simulink library "lib6DOFDerivativeOfEquations"  (R2020b)
settings: Solver=VariableStepAuto  StartTime=0.0  StopTime=10.0  RelTol=1e-3
undefined symbols (not defined in the file): data
settings Model: Creator=caatay  LastModifiedBy=caatay

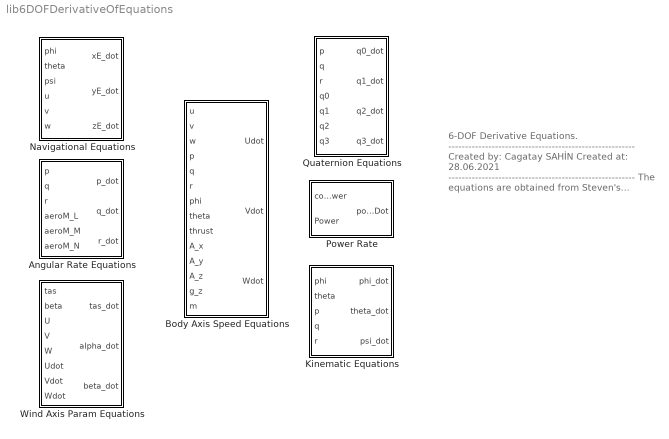
== system lib6DOFDerivativeOfEquations ==
  note: 6-DOF Derivative Equations.
      | --------------------------------------------------------
      | Created by: Cagatay SAHİN
      | Created at: 28.06.2021
      | --------------------------------------------------------
      | The equations are obtained from
      | Steven's textbook.
      | The reference book can be found in
      | "references folder".
      | --------------------------------------------------------
      | for question:
      | cagataysahin44@gmail.com
  Angular Rate Equations : Subsystem  mask(Equation of Motion - Derivative Equations of Motion - CAME (Angular Rate) Equations.){I_xx=data.acSpec.inertia.I_xx, I_yy=data.acSpec.inertia.I_yy, I_zz=data.acSpec.inertia.I_zz, I_xz=data.acSpec.inertia.I_xz, h_x=data.engine.specs.angMom.h_x}
      mask prompts: I_xx "Inertia on X-axis"; I_yy "Inertia on Y-axis"; I_zz "Inertia on Z-axis"; I_xz "Inertia on XZ-axis"; h_x "Angular Momentum on X-axis"
      mask help: Aircraft Conversation of Angular Momentum Equation which calculates angular rates.
      mask Help:
      | Aircraft Conversation of Angular Momentum Equation which calculates angular rates which using moment and state information as an input.
      | -------------------------------------------------------------------------------------------------------------------------------------------------
      | Inputs of this block:
      | 	Body Axis Speed: U, V, W information [ft/s].
      | 	Body Axis Moments: M_l, M_M, M_N information
      | Outputs of this block:
      | 	Ang. Rates Der.: Derivative of Angular Rates [rad/sec^2].
      | -------------------------------------------------------------------------------------------------------------------------------------------------
      | Equations that in this block can be found in Steven's textbook. This textbook is in "literature" subfolder.
      | for question: "cagataysahin44@gmail.com".
      mask Display:
      | port_label('input',1,'p','texmode','on');
      | port_label('input',2,'q','texmode','on');
      | port_label('input',3,'r','texmode','on');
      | port_label('input',4,'M_{L}','texmode','on');
      | port_label('input',5,'M_{M}','texmode','on');
      | port_label('input',6,'M_{N}','texmode','on');
      | 
      | port_label('output',1,'p_{der}','texmode','on');
      | port_label('output',2,'q_{der}','texmode','on');
      | port_label('output',3,'r_{der}','texmode','on');
  Body Axis Speed Equations : Subsystem  mask(EOM Model - Derivative Equation of Motion - Body Axis Speed Equations){}
      mask help: Aircraft body axis speeds calculation equations.
      mask Help:
      | This block can calculate aircraft's body axis speeds with using state, thrust, force and gravity information.
      | -------------------------------------------------------------------------------------------------------------------------------------------------
      | Inputs of this block:
      | 	Euler Angles: Roll, Pitch information [rad].
      | 	Body Axis Speed: U, V, W information [ft/s].
      | 	T: Thrust information [lbf].
      | 	A_{i}: Aerodynamic force information [lbf].
      | 	g: gravity information [ft/sec^2].
      | 	m: Aircraft Mass [slug].
      | Outputs of this block:
      | 	Body Axis Speed Ders. Derivative of body axis speeds [ft/sec^2].
      | -------------------------------------------------------------------------------------------------------------------------------------------------
      | Equations that in this block can be found in Steven's textbook. This textbook is in "literature" subfolder.
      | for question: "cagataysahin44@gmail.com".
      mask Display:
      | port_label('input',1,'U','texmode','on');
      | port_label('input',2,'V','texmode','on');
      | port_label('input',3,'W','texmode','on');
      | port_label('input',4,'p','texmode','on');
      | port_label('input',5,'q','texmode','on');
      | port_label('input',6,'r','texmode','on');
      | port_label('input',7,'\phi','texmode','on');
      | port_label('input',8,'\theta','texmode','on');
      | port_label('input',9,'T','texmode','on');
      | port_label('input',10,'A_{x}','texmode','on');
      | port_label('input',11,'A_{y}','texmode','on');
      | port_label('input',12,'A_{z}','texmode','on');
      | port_label('input',13,'g_{z}','texmode','on');
      | port_label('input',14,'m','texmode','on');
      | 
      | port_label('output',1,'U_{der}','texmode','on');
      | port_label('output',2,'V_{der}','texmode','on');
      | port_label('output',3,'W_{der}','texmode','on');
  Kinematic Equations : Subsystem  mask(Equation of Motion - Derivative Equation of Motion - Kinematic Equation for Euler Angles.){}
      mask help: Aircraft kinematic equtions which is in Euler Angles form.
      mask Help:
      | This block can calculate aircaft's kinematic parameters in Euler Angles form.
      | -------------------------------------------------------------------------------------------------------------------------------------------------
      | Inputs of this block:
      | 	Euler Angles: Roll, Pitch, information [rad].
      | 	Body Axis Angular Rates: p, q, r information [rad/s].
      | Outputs of this block:
      | 	Euler Angles Ders: Derivative of Euler Angles.
      | -------------------------------------------------------------------------------------------------------------------------------------------------
      | Equations that in this block can be found in Steven's textbook. This textbook is in "literature" subfolder.
      | for question: "cagataysahin44@gmail.com".
      mask Display:
      | port_label('input',1,'\phi','texmode','on');
      | port_label('input',2,'\theta','texmode','on');
      | port_label('input',3,'p','texmode','on');
      | port_label('input',4,'q','texmode','on');
      | port_label('input',5,'r','texmode','on');
      | 
      | port_label('output',1,'\phi_{der}','texmode','on');
      | port_label('output',2,'\theta_{der}','texmode','on');
      | port_label('output',3,'\psi_{der}','texmode','on');
  Navigational Equations : Subsystem  mask(EOM Model - Derivative Equations - Navigational Equations){}
      mask help: Aircraft navigational equations which is known as flight path.
      mask Help:
      | This block can calculate aircaft's flight path information with using state inputs.
      | -------------------------------------------------------------------------------------------------------------------------------------------------
      | Inputs of this block:
      | 	Euler Angles: Roll, Pitch, Yaw information [rad].
      | 	Body Axis Speed: U, V, W information [ft/s].
      | Outputs of this block:
      | 	p_{e}: Derivative of position of aircraft in NED Coordinate System [ft].
      | -------------------------------------------------------------------------------------------------------------------------------------------------
      | Equations that in this block can be found in Steven's textbook. This textbook is in "literature" subfolder.
      | for question: "cagataysahin44@gmail.com".
      mask Display:
      | port_label('input',1,'\phi','texmode','on');
      | port_label('input',2,'\theta','texmode','on');
      | port_label('input',3,'\psi','texmode','on');
      | port_label('input',4,'u','texmode','on');
      | port_label('input',5,'v','texmode','on');
      | port_label('input',6,'w','texmode','on');
      | 
      | port_label('output',1,'x_{e_{der}}','texmode','on');
      | port_label('output',2,'y_{e_{der}}','texmode','on');
      | port_label('output',3,'z_{e_{der}}','texmode','on');
  Power Rate : Subsystem  mask(EOM Model - Derivative of Equation of Motion - Power Rate Calculation){}
      mask help: Derivative of power calculation with using actual power information as a state and commanded power information from throttle command.
      mask Help:
      | This block can calculate aircaft's power derivative equation.
      | -------------------------------------------------------------------------------------------------------------------------------------------------
      | Inputs of this block:
      | 	cmdPow: Commanded Power [hp].
      | 	actPow: Actual Power [hp].
      | Outputs of this block:
      | 	powDot: Derivative of Power [hp/s]
      | -------------------------------------------------------------------------------------------------------------------------------------------------
      | Equations that in this block can be found in Steven's textbook. This textbook is in "literature" subfolder.
      | for question: "cagataysahin44@gmail.com".
      mask Display:
      | port_label('input',1,'Pow_{cmd}','texmode','on');
      | port_label('input',2,'Pow_{act}','texmode','on');
      | 
      | port_label('output',1,'der_{Pow_{act}}','texmode','on');
  Quaternion Equations : Subsystem  mask(Equation of Motion - Derivative Equation of Motion - Kinematic Equation for Quaternion Angles.){}
      mask help: Aircraft kinematic equtions which is in quaternion angles form.
      mask Help:
      | This block can calculate aircaft's kinematic parameters in quaternion angles form.
      | -------------------------------------------------------------------------------------------------------------------------------------------------
      | Inputs of this block:
      | 	Quaternion Angles: q0, q1, q2, q3, information [rad].
      | 	Body Axis Angular Rates: p, q, r information [rad/s].
      | Outputs of this block:
      | 	Quaternion Angles Ders: Derivative of Quaternion Angles.
      | -------------------------------------------------------------------------------------------------------------------------------------------------
      | Equations that in this block can be found in Steven's textbook. This textbook is in "literature" subfolder.
      | for question: "cagataysahin44@gmail.com".
      mask Display:
      | port_label('input',1,'p','texmode','on');
      | port_label('input',2,'q','texmode','on');
      | port_label('input',3,'r','texmode','on');
      | port_label('input',4,'q_{0}','texmode','on');
      | port_label('input',5,'q_{1}','texmode','on');
      | port_label('input',6,'q_{2}','texmode','on');
      | port_label('input',7,'q_{3}','texmode','on');
      | 
      | port_label('output',1,'q_{1_{der}}','texmode','on');
      | port_label('output',2,'q_{2_{der}}','texmode','on');
      | port_label('output',3,'q_{3_{der}}','texmode','on');
      | port_label('output',4,'q_{4_{der}}','texmode','on');
  Wind Axis Param Equations : Subsystem  mask(EOM Model - Derivative of Equation of Motion - Wind Axis Paramater Equations.){}
      mask help: Aircraft wind parameter information calculation which is angle of attack, angle of sideslip and true airspeed.
      mask Help:
      | This block can calculate aircaft's wind parameters which using state inputs.
      | -------------------------------------------------------------------------------------------------------------------------------------------------
      | Inputs of this block:
      | 	Wind Params: True airspeed, AoA and AoS [ft/s, rad].
      | 	Body Speeds: U, V, W information [ft/s].
      | 	Body Speed Ders: U, V, W derivative information [ft/sec^2].
      | Outputs of this block:
      | 	Wind Param Ders: Derivative information of wind parameters. [ft/sec^2, rad/sec].
      | -------------------------------------------------------------------------------------------------------------------------------------------------
      | Equations that in this block can be found in Steven's textbook. This textbook is in "literature" subfolder.
      | for question: "cagataysahin44@gmail.com".
      mask Display:
      | port_label('input',1,'V_{tas}','texmode','on');
      | port_label('input',2,'\beta','texmode','on');
      | port_label('input',3,'U','texmode','on');
      | port_label('input',4,'V','texmode','on');
      | port_label('input',5,'W','texmode','on');
      | port_label('input',6,'U_{der}','texmode','on');
      | port_label('input',7,'V_{der}','texmode','on');
      | port_label('input',8,'W_{der}','texmode','on');
      | 
      | port_label('output',1,'V_{tas_{der}}','texmode','on');
      | port_label('output',2,'\alpha_{der}','texmode','on');
      | port_label('output',3,'\beta_{der}','texmode','on');

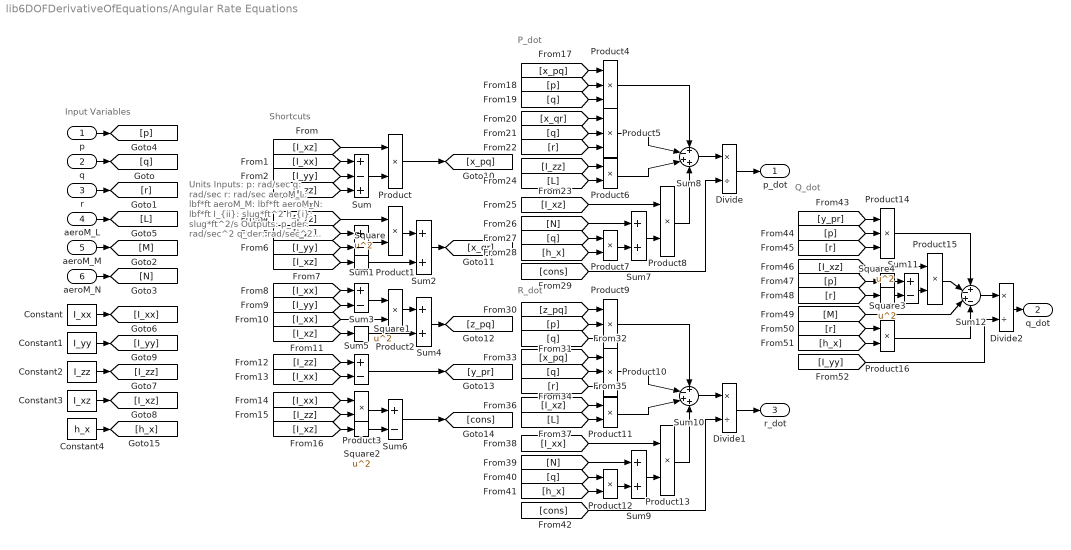
== system lib6DOFDerivativeOfEquations/Angular Rate Equations ==
  note: Q_dot
  note: P_dot
  note: Shortcuts
  note: Units
      | Inputs:
      | p: rad/sec
      | q: rad/sec
      | r: rad/sec
      | aeroM_L: lbf*ft
      | aeroM_M: lbf*ft
      | aeroM_N: lbf*ft
      | I_{ii}: slug*ft^2
      | h_{i}: slug*ft^2/s
      | Outputs:
      | p_der: rad/sec^2
      | q_der: rad/sec^2
      | r_der: rad/sec^2
  note: Input Variables
  note: R_dot
  p : Inport
  q : Inport  Port=2
  r : Inport  Port=3
  aeroM_L : Inport  Port=4
  aeroM_M : Inport  Port=5
  aeroM_N : Inport  Port=6
  Constant : Constant  Value=I_xx
  Constant1 : Constant  Value=I_yy
  Constant2 : Constant  Value=I_zz
  Constant3 : Constant  Value=I_xz
  Constant4 : Constant  Value=h_x
  Divide : Product  Inputs=*/
  Divide1 : Product  Inputs=*/
  Divide2 : Product  Inputs=*/
  Product{,1..3,6..8,11..13,15..16} (12 alike) : Product
  Product{4..5,9..10,14} (5 alike) : Product  Inputs=3
  Square{,1..4} (5 alike) : Math  Operator=square  SignedPower=on  SaturateOnIntegerOverflow=on
  Sum : Sum  Inputs=+-+
  Sum{1,3,5..6,11} (5 alike) : Sum  Inputs=+-
  Sum10 : Sum  Inputs=+-++
  Sum12 : Sum  Inputs=+-+-
  Sum{2,4,7,9} (4 alike) : Sum
  Sum8 : Sum  Inputs=+-++
  p_dot : Outport  VectorParamsAs1DForOutWhenUnconnected=off
  q_dot : Outport  Port=2  VectorParamsAs1DForOutWhenUnconnected=off
  r_dot : Outport  Port=3  VectorParamsAs1DForOutWhenUnconnected=off
  wires:
  p/1 -> [p]
  q/1 -> [q]
  r/1 -> [r]
  aeroM_L/1 -> [L]
  aeroM_M/1 -> [M]
  aeroM_N/1 -> [N]
  Constant/1 -> [I_xx]
  Constant3/1 -> [I_xz]
  Constant2/1 -> [I_zz]
  Constant1/1 -> [I_yy]
  [I_xx] -> Sum/1
  [I_zz] -> Sum/3
  [I_yy] -> Sum/2
  [I_xz] -> Product/1
  Sum/1 -> Product/2
  Product/1 -> [x_pq]
  [I_xz] -> Square/1
  [I_zz] -> Sum1/1
  [I_yy] -> Sum1/2
  Sum1/1 -> Product1/2
  [I_zz] -> Product1/1
  Product1/1 -> Sum2/1
  Square/1 -> Sum2/2
  Sum2/1 -> [x_qr]
  [I_xz] -> Square1/1
  [I_xx] -> Product2/2
  [I_yy] -> Sum3/2
  [I_xx] -> Sum3/1
  Sum3/1 -> Product2/1
  Product2/1 -> Sum4/1
  Square1/1 -> Sum4/2
  Sum4/1 -> [z_pq]
  [I_zz] -> Sum5/1
  [I_xx] -> Sum5/2
  Sum5/1 -> [y_pr]
  [I_zz] -> Product3/2
  [I_xx] -> Product3/1
  [I_xz] -> Square2/1
  Product3/1 -> Sum6/1
  Square2/1 -> Sum6/2
  Sum6/1 -> [cons]
  Constant4/1 -> [h_x]
  [x_pq] -> Product4/1
  [p] -> Product4/2
  [q] -> Product4/3
  [q] -> Product5/2
  [x_qr] -> Product5/1
  [r] -> Product5/3
  [I_zz] -> Product6/1
  [L] -> Product6/2
  [q] -> Product7/1
  [h_x] -> Product7/2
  [N] -> Sum7/1
  [I_xz] -> Product8/1
  Product7/1 -> Sum7/2
  Sum7/1 -> Product8/2
  Product6/1 -> Sum8/3
  Product5/1 -> Sum8/2
  Product4/1 -> Sum8/1
  Product8/1 -> Sum8/4
  Sum8/1 -> Divide/1
  Divide/1 -> p_dot/1
  [cons] -> Divide/2
  Product12/1 -> Sum9/2
  Sum9/1 -> Product13/2
  [N] -> Sum9/1
  Sum10/1 -> Divide1/1
  [q] -> Product12/1
  Product13/1 -> Sum10/4
  Product9/1 -> Sum10/1
  [I_xz] -> Product11/1
  [h_x] -> Product12/2
  Divide1/1 -> r_dot/1
  [x_pq] -> Product10/1
  [q] -> Product10/2
  [I_xx] -> Product13/1
  [z_pq] -> Product9/1
  [q] -> Product9/3
  [L] -> Product11/2
  Product10/1 -> Sum10/2
  [p] -> Product9/2
  [cons] -> Divide1/2
  [r] -> Product10/3
  Product11/1 -> Sum10/3
  [y_pr] -> Product14/1
  [p] -> Product14/2
  Product14/1 -> Sum12/1
  [r] -> Product14/3
  [p] -> Square3/1
  [r] -> Square4/1
  Square3/1 -> Sum11/1
  Square4/1 -> Sum11/2
  [I_xz] -> Product15/1
  Sum11/1 -> Product15/2
  [r] -> Product16/1
  [h_x] -> Product16/2
  [M] -> Sum12/3
  Product15/1 -> Sum12/2
  Product16/1 -> Sum12/4
  Sum12/1 -> Divide2/1
  [I_yy] -> Divide2/2
  Divide2/1 -> q_dot/1

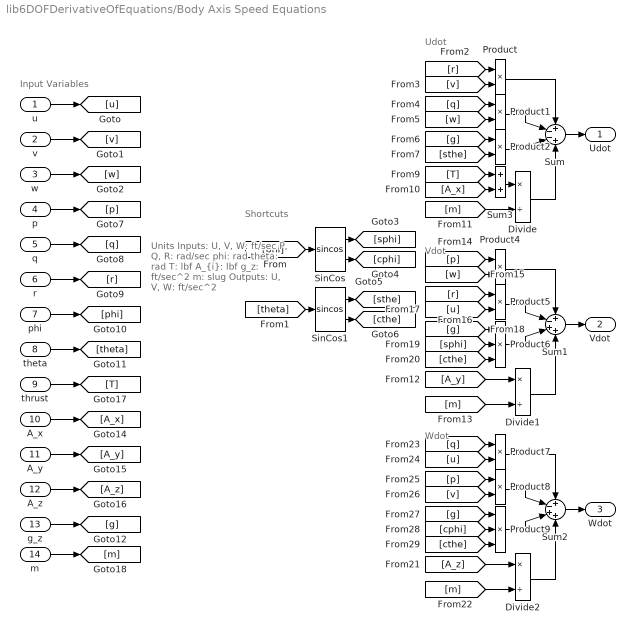
== system lib6DOFDerivativeOfEquations/Body Axis Speed Equations ==
  note: Vdot
  note: Input Variables
  note: Wdot
  note: Udot
  note: Shortcuts
  note: Units
      | Inputs:
      | U, V, W: ft/sec
      | P, Q, R: rad/sec
      | phi: rad
      | theta: rad
      | T: lbf
      | A_{i}: lbf
      | g_z: ft/sec^2
      | m: slug
      | Outputs:
      | U, V, W: ft/sec^2
  u : Inport
  v : Inport  Port=2
  w : Inport  Port=3
  p : Inport  Port=4
  q : Inport  Port=5
  r : Inport  Port=6
  phi : Inport  Port=7
  theta : Inport  Port=8
  thrust : Inport  Port=9
  A_x : Inport  Port=10
  A_y : Inport  Port=11
  A_z : Inport  Port=12
  g_z : Inport  Port=13
  m : Inport  Port=14
  Divide : Product  Inputs=*/
  Divide1 : Product  Inputs=*/
  Divide2 : Product  Inputs=*/
  Product{,1..2,4..5,7..8} (7 alike) : Product
  Product6 : Product  Inputs=3
  Product9 : Product  Inputs=3
  SinCos : Trigonometry  Operator=sincos
  SinCos1 : Trigonometry  Operator=sincos
  Sum : Sum  Inputs=+--+
  Sum1 : Sum  Inputs=+-++
  Sum2 : Sum  Inputs=+-++
  Sum3 : Sum
  Udot : Outport  VectorParamsAs1DForOutWhenUnconnected=off
  Vdot : Outport  Port=2  VectorParamsAs1DForOutWhenUnconnected=off
  Wdot : Outport  Port=3  VectorParamsAs1DForOutWhenUnconnected=off
  wires:
  u/1 -> [u]
  SinCos/1 -> [sphi]
  v/1 -> [v]
  [phi] -> SinCos/1
  SinCos1/1 -> [sthe]
  SinCos/2 -> [cphi]
  SinCos1/2 -> [cthe]
  [theta] -> SinCos1/1
  [r] -> Product/1
  [v] -> Product/2
  w/1 -> [w]
  p/1 -> [p]
  r/1 -> [r]
  q/1 -> [q]
  theta/1 -> [theta]
  phi/1 -> [phi]
  [w] -> Product1/2
  [q] -> Product1/1
  g_z/1 -> [g]
  [sthe] -> Product2/2
  [g] -> Product2/1
  A_x/1 -> [A_x]
  thrust/1 -> [T]
  [A_x] -> Sum3/2
  [T] -> Sum3/1
  m/1 -> [m]
  Sum/1 -> Udot/1
  Sum3/1 -> Divide/1
  [m] -> Divide/2
  Divide/1 -> Sum/4
  Product1/1 -> Sum/2
  Product/1 -> Sum/1
  [w] -> Product4/2
  [p] -> Product4/1
  [g] -> Product6/1
  [A_y] -> Divide1/1
  Sum1/1 -> Vdot/1
  Product4/1 -> Sum1/1
  [m] -> Divide1/2
  Product6/1 -> Sum1/3
  Product5/1 -> Sum1/2
  [r] -> Product5/1
  [u] -> Product5/2
  Divide1/1 -> Sum1/4
  [sphi] -> Product6/2
  [cthe] -> Product6/3
  [A_z] -> Divide2/1
  Divide2/1 -> Sum2/4
  [p] -> Product8/1
  [cphi] -> Product9/2
  Product9/1 -> Sum2/3
  [q] -> Product7/1
  [m] -> Divide2/2
  Product8/1 -> Sum2/2
  [g] -> Product9/1
  [v] -> Product8/2
  [u] -> Product7/2
  Product7/1 -> Sum2/1
  [cthe] -> Product9/3
  Sum2/1 -> Wdot/1
  A_y/1 -> [A_y]
  A_z/1 -> [A_z]
  Product2/1 -> Sum/3

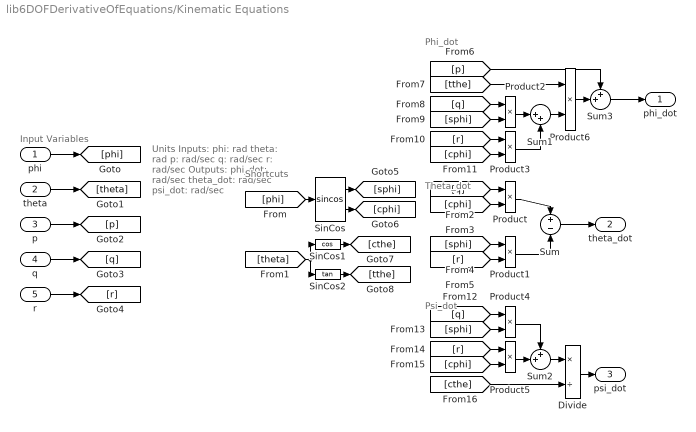
== system lib6DOFDerivativeOfEquations/Kinematic Equations ==
  note: Theta_dot
  note: Units
      | Inputs:
      | phi: rad
      | theta: rad
      | p: rad/sec
      | q: rad/sec
      | r: rad/sec
      | Outputs:
      | phi_dot: rad/sec
      | theta_dot: rad/sec
      | psi_dot: rad/sec
  note: Input Variables
  note: Shortcuts
  note: Phi_dot
  note: Psi_dot
  "phi " : Inport
  theta : Inport  Port=2
  p : Inport  Port=3
  q : Inport  Port=4
  r : Inport  Port=5
  Divide : Product  Inputs=*/
  Product{,1..6} (7 alike) : Product
  SinCos : Trigonometry  Operator=sincos
  SinCos1 : Trigonometry  Operator=cos
  SinCos2 : Trigonometry  Operator=tan
  Sum : Sum  Inputs=+-
  Sum1 : Sum  Inputs=|++
  Sum2 : Sum  Inputs=++|
  Sum3 : Sum  Inputs=++|
  phi_dot : Outport  VectorParamsAs1DForOutWhenUnconnected=off
  theta_dot : Outport  Port=2  VectorParamsAs1DForOutWhenUnconnected=off
  psi_dot : Outport  Port=3  VectorParamsAs1DForOutWhenUnconnected=off
  wires:
  "phi "/1 -> [phi]
  p/1 -> [p]
  theta/1 -> [theta]
  q/1 -> [q]
  r/1 -> [r]
  SinCos2/1 -> [tthe]
  SinCos1/1 -> [cthe]
  SinCos/1 -> [sphi]
  SinCos/2 -> [cphi]
  [phi] -> SinCos/1
  [theta] -> SinCos1/1, SinCos2/1
  [q] -> Product/1
  [cphi] -> Product/2
  [sphi] -> Product1/1
  [r] -> Product1/2
  Product/1 -> Sum/1
  Product1/1 -> Sum/2
  Sum/1 -> theta_dot/1
  [q] -> Product2/1
  [sphi] -> Product2/2
  [tthe] -> Product6/1
  [cphi] -> Product3/2
  [r] -> Product3/1
  Product2/1 -> Sum1/1
  [p] -> Sum3/1
  Product3/1 -> Sum1/2
  Sum3/1 -> phi_dot/1
  [cphi] -> Product5/2
  [r] -> Product5/1
  [q] -> Product4/1
  [sphi] -> Product4/2
  Product5/1 -> Sum2/2
  Product4/1 -> Sum2/1
  Sum2/1 -> Divide/1
  [cthe] -> Divide/2
  Divide/1 -> psi_dot/1
  Sum1/1 -> Product6/2
  Product6/1 -> Sum3/2

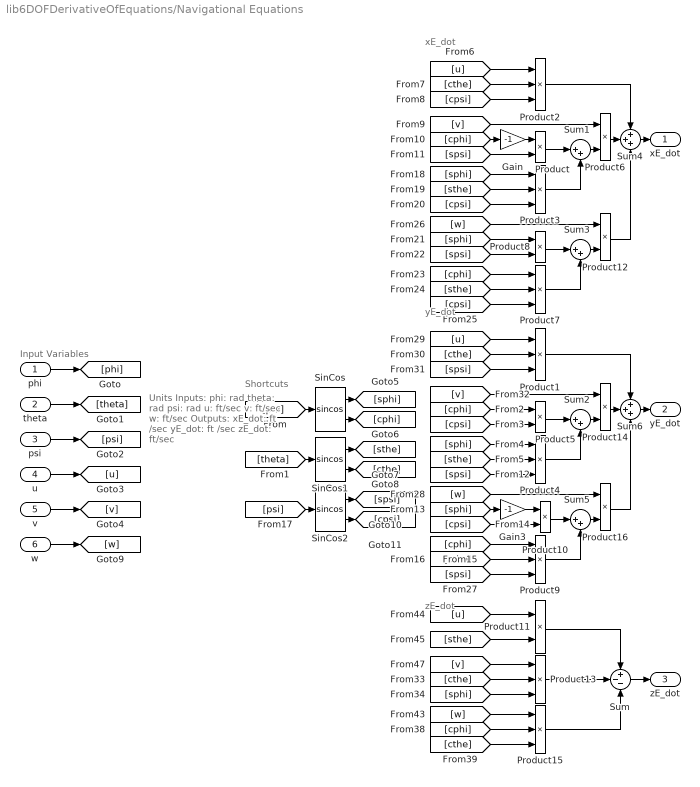
== system lib6DOFDerivativeOfEquations/Navigational Equations ==
  note: xE_dot
  note: Shortcuts
  note: Input Variables
  note: Units
      | Inputs:
      | phi: rad
      | theta: rad
      | psi: rad
      | u: ft/sec
      | v: ft/sec
      | w: ft/sec
      | Outputs:
      | xE_dot: ft /sec
      | yE_dot: ft /sec
      | zE_dot: ft/sec
  note: yE_dot
  note: zE_dot
  "phi " : Inport
  theta : Inport  Port=2
  psi : Inport  Port=3
  u : Inport  Port=4
  v : Inport  Port=5
  w : Inport  Port=6
  Gain : Gain  Gain=-1
  Gain3 : Gain  Gain=-1
  Product{,5..6,8,10..12,14,16} (9 alike) : Product
  Product{1..4,7,9,13,15} (8 alike) : Product  Inputs=3
  SinCos : Trigonometry  Operator=sincos
  SinCos1 : Trigonometry  Operator=sincos
  SinCos2 : Trigonometry  Operator=sincos
  Sum : Sum  Inputs=+--
  Sum{1..3,5} (4 alike) : Sum  Inputs=|++
  Sum4 : Sum  Inputs=+++
  Sum6 : Sum  Inputs=+++
  xE_dot : Outport  VectorParamsAs1DForOutWhenUnconnected=off
  yE_dot : Outport  Port=2  VectorParamsAs1DForOutWhenUnconnected=off
  zE_dot : Outport  Port=3  VectorParamsAs1DForOutWhenUnconnected=off
  wires:
  v/1 -> [v]
  theta/1 -> [theta]
  "phi "/1 -> [phi]
  [phi] -> SinCos/1
  SinCos/2 -> [cphi]
  u/1 -> [u]
  psi/1 -> [psi]
  SinCos/1 -> [sphi]
  w/1 -> [w]
  SinCos1/2 -> [cthe]
  [theta] -> SinCos1/1
  [psi] -> SinCos2/1
  SinCos2/2 -> [cpsi]
  SinCos2/1 -> [spsi]
  SinCos1/1 -> [sthe]
  [u] -> Product2/1
  [cthe] -> Product2/2
  [cpsi] -> Product2/3
  [cphi] -> Gain/1
  [sthe] -> Product3/2
  [cpsi] -> Product3/3
  [sphi] -> Product3/1
  [spsi] -> Product/2
  [v] -> Product6/1
  Gain/1 -> Product/1
  Product/1 -> Sum1/1
  Product3/1 -> Sum1/2
  [spsi] -> Product8/2
  [w] -> Product12/1
  Product7/1 -> Sum3/2
  [cphi] -> Product7/1
  [cpsi] -> Product7/3
  [sthe] -> Product7/2
  [sphi] -> Product8/1
  Product8/1 -> Sum3/1
  Product2/1 -> Sum4/1
  Sum1/1 -> Product6/2
  Sum4/1 -> xE_dot/1
  Product9/1 -> Sum5/2
  Product1/1 -> Sum6/1
  Sum6/1 -> yE_dot/1
  [u] -> Product1/1
  [cthe] -> Product1/2
  [spsi] -> Product1/3
  [sthe] -> Product4/2
  Gain3/1 -> Product10/1
  Product5/1 -> Sum2/1
  Product10/1 -> Sum5/1
  [cphi] -> Product5/1
  [spsi] -> Product9/3
  [cpsi] -> Product10/2
  [w] -> Product16/1
  [sthe] -> Product9/2
  [sphi] -> Gain3/1
  Product4/1 -> Sum2/2
  [cphi] -> Product9/1
  [cpsi] -> Product5/2
  [sphi] -> Product4/1
  [spsi] -> Product4/3
  [v] -> Product13/1
  [u] -> Product11/1
  [sthe] -> Product11/2
  [cphi] -> Product15/2
  [cthe] -> Product13/2
  [cthe] -> Product15/3
  [w] -> Product15/1
  [sphi] -> Product13/3
  Product11/1 -> Sum/1
  Product13/1 -> Sum/2
  Product15/1 -> Sum/3
  Sum/1 -> zE_dot/1
  Product6/1 -> Sum4/2
  Sum3/1 -> Product12/2
  Product12/1 -> Sum4/3
  Sum2/1 -> Product14/2
  Product14/1 -> Sum6/2
  [v] -> Product14/1
  Sum5/1 -> Product16/2
  Product16/1 -> Sum6/3

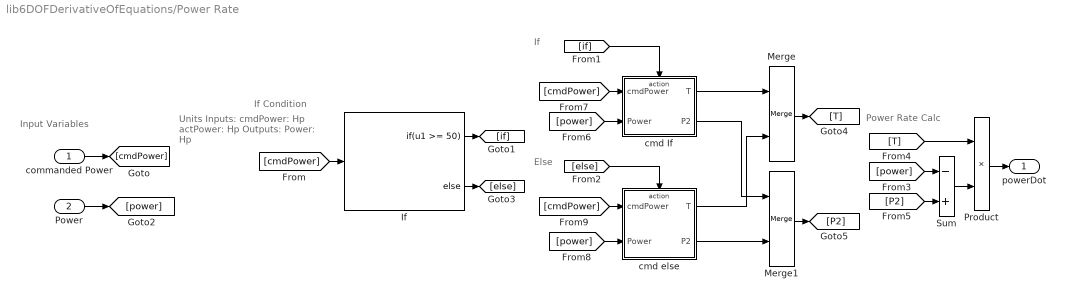
== system lib6DOFDerivativeOfEquations/Power Rate ==
  note: Power Rate Calc
  note: Input Variables
  note: Units
      | Inputs:
      | cmdPower: Hp
      | actPower: Hp
      | Outputs:
      | Power: Hp
  note: If Condition
  note: If
  note: Else
  commanded Power : Inport
  Power : Inport  Port=2
  If : If  IfExpression=u1 >= 50
  Merge : Merge
  Merge1 : Merge
  Product : Product
  Sum : Sum  Inputs=-+
  cmd If : Subsystem  TreatAsAtomicUnit=on
  cmd else : Subsystem  TreatAsAtomicUnit=on
  powerDot : Outport  VectorParamsAs1DForOutWhenUnconnected=off
  wires:
  commanded Power/1 -> [cmdPower]
  [cmdPower] -> If/1
  If/1 -> [if]
  If/2 -> [else]
  [if] -> cmd If/Action
  [else] -> cmd else/Action
  Merge/1 -> [T]
  Merge1/1 -> [P2]
  [power] -> Sum/1
  [P2] -> Sum/2
  Sum/1 -> Product/2
  [T] -> Product/1
  Product/1 -> powerDot/1
  [power] -> cmd If/2(Power)
  [cmdPower] -> cmd If/1(cmdPower)
  [power] -> cmd else/2(Power)
  [cmdPower] -> cmd else/1(cmdPower)
  cmd else/2(P2) -> Merge1/2
  cmd If/1(T) -> Merge/1
  cmd If/2(P2) -> Merge1/1
  cmd else/1(T) -> Merge/2
  Power/1 -> [power]

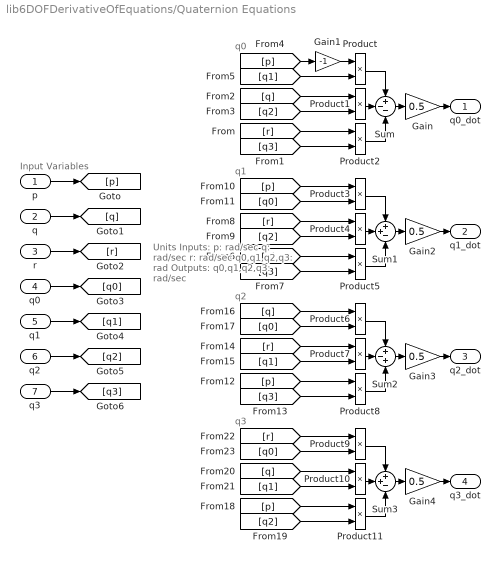
== system lib6DOFDerivativeOfEquations/Quaternion Equations ==
  note: q0
  note: Units
      | Inputs:
      | p: rad/sec
      | q: rad/sec
      | r: rad/sec
      | q0,q1,q2,q3: rad
      | Outputs:
      | q0,q1,q2,q3: rad/sec
  note: Input Variables
  note: q1
  note: q2
  note: q3
  "p " : Inport
  q : Inport  Port=2
  r : Inport  Port=3
  q0 : Inport  Port=4
  q1 : Inport  Port=5
  q2 : Inport  Port=6
  q3 : Inport  Port=7
  Gain{,2..4} (4 alike) : Gain  Gain=0.5
  Gain1 : Gain  Gain=-1
  Product{,1..11} (12 alike) : Product
  Sum : Sum  Inputs=+--
  Sum1 : Sum  Inputs=++-
  Sum2 : Sum  Inputs=+-+
  Sum3 : Sum  Inputs=++-
  q0_dot : Outport  VectorParamsAs1DForOutWhenUnconnected=off
  q1_dot : Outport  Port=2  VectorParamsAs1DForOutWhenUnconnected=off
  q2_dot : Outport  Port=3  VectorParamsAs1DForOutWhenUnconnected=off
  q3_dot : Outport  Port=4  VectorParamsAs1DForOutWhenUnconnected=off
  wires:
  r/1 -> [r]
  q/1 -> [q]
  "p "/1 -> [p]
  q2/1 -> [q2]
  q1/1 -> [q1]
  q3/1 -> [q3]
  q0/1 -> [q0]
  Product/1 -> Sum/1
  [q1] -> Product/2
  [q2] -> Product1/2
  Sum/1 -> Gain/1
  [q3] -> Product2/2
  [p] -> Gain1/1
  [r] -> Product2/1
  [q] -> Product1/1
  Gain1/1 -> Product/1
  Gain/1 -> q0_dot/1
  Product1/1 -> Sum/2
  Product2/1 -> Sum/3
  Product4/1 -> Sum1/2
  Gain2/1 -> q1_dot/1
  [p] -> Product3/1
  [r] -> Product4/1
  [q3] -> Product5/2
  Sum1/1 -> Gain2/1
  [q2] -> Product4/2
  Product3/1 -> Sum1/1
  [q] -> Product5/1
  Product5/1 -> Sum1/3
  [q0] -> Product3/2
  Product7/1 -> Sum2/2
  Gain3/1 -> q2_dot/1
  [q] -> Product6/1
  [r] -> Product7/1
  [q3] -> Product8/2
  Sum2/1 -> Gain3/1
  [q1] -> Product7/2
  Product6/1 -> Sum2/1
  [p] -> Product8/1
  Product8/1 -> Sum2/3
  [q0] -> Product6/2
  Product10/1 -> Sum3/2
  Gain4/1 -> q3_dot/1
  [r] -> Product9/1
  [q] -> Product10/1
  [q2] -> Product11/2
  Sum3/1 -> Gain4/1
  [q1] -> Product10/2
  Product9/1 -> Sum3/1
  [p] -> Product11/1
  Product11/1 -> Sum3/3
  [q0] -> Product9/2

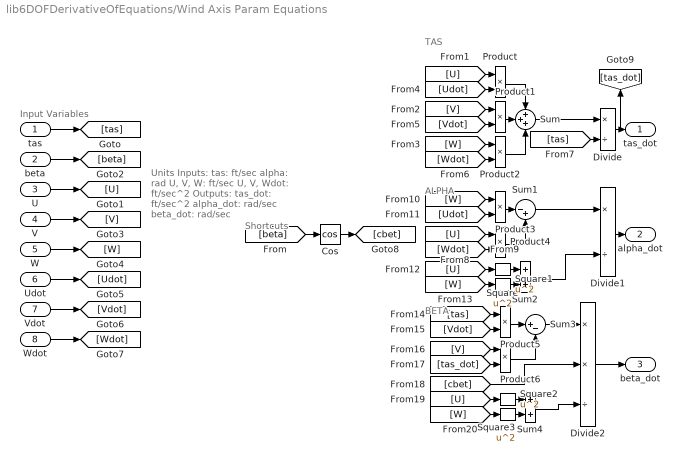
== system lib6DOFDerivativeOfEquations/Wind Axis Param Equations ==
  note: Units
      | Inputs:
      | tas: ft/sec
      | alpha: rad
      | U, V, W: ft/sec
      | U, V, Wdot: ft/sec^2
      | Outputs:
      | tas_dot: ft/sec^2
      | alpha_dot: rad/sec
      | beta_dot: rad/sec
  note: Shortcuts
  note: BETA
  note: Input Variables
  note: ALPHA
  note: TAS
  tas : Inport
  beta : Inport  Port=2
  U : Inport  Port=3
  V : Inport  Port=4
  W : Inport  Port=5
  Udot : Inport  Port=6
  Vdot : Inport  Port=7
  Wdot : Inport  Port=8
  Cos : Trigonometry  Operator=cos
  Divide : Product  Inputs=*/
  Divide1 : Product  Inputs=*/
  Divide2 : Product  Inputs=**/
  Product{,1..6} (7 alike) : Product
  Square{,1..3} (4 alike) : Math  Operator=square  SignedPower=on  SaturateOnIntegerOverflow=on
  Sum : Sum  Inputs=+++
  Sum1 : Sum  Inputs=|-+
  Sum2 : Sum
  Sum3 : Sum  Inputs=|+-
  Sum4 : Sum
  tas_dot : Outport  VectorParamsAs1DForOutWhenUnconnected=off
  alpha_dot : Outport  Port=2  VectorParamsAs1DForOutWhenUnconnected=off
  beta_dot : Outport  Port=3  VectorParamsAs1DForOutWhenUnconnected=off
  wires:
  beta/1 -> [beta]
  tas/1 -> [tas]
  U/1 -> [U]
  V/1 -> [V]
  W/1 -> [W]
  Udot/1 -> [Udot]
  Vdot/1 -> [Vdot]
  Wdot/1 -> [Wdot]
  [beta] -> Cos/1
  Cos/1 -> [cbet]
  [U] -> Product/1
  [Wdot] -> Product2/2
  [W] -> Product2/1
  [Vdot] -> Product1/2
  [V] -> Product1/1
  [Udot] -> Product/2
  Product1/1 -> Sum/2
  Product/1 -> Sum/1
  Product2/1 -> Sum/3
  [tas] -> Divide/2
  Sum/1 -> Divide/1
  Square1/1 -> Sum2/2
  [W] -> Product3/1
  Divide1/1 -> alpha_dot/1
  Square/1 -> Sum2/1
  Product4/1 -> Sum1/2
  Sum1/1 -> Divide1/1
  [W] -> Square1/1
  Sum2/1 -> Divide1/2
  [U] -> Product4/1
  [Wdot] -> Product4/2
  [U] -> Square/1
  Product3/1 -> Sum1/1
  [Udot] -> Product3/2
  Divide/1 -> tas_dot/1, [tas_dot]
  Product6/1 -> Sum3/2
  Square2/1 -> Sum4/1
  Square3/1 -> Sum4/2
  [W] -> Square3/1
  [U] -> Square2/1
  Divide2/1 -> beta_dot/1
  Sum4/1 -> Divide2/3
  [V] -> Product6/1
  Product5/1 -> Sum3/1
  [tas_dot] -> Product6/2
  [cbet] -> Divide2/2
  [tas] -> Product5/1
  [Vdot] -> Product5/2
  Sum3/1 -> Divide2/1

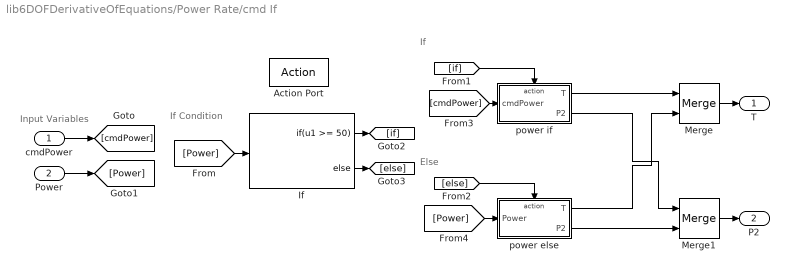
== system lib6DOFDerivativeOfEquations/Power Rate/cmd If ==
  note: Input Variables
  note: If
  note: Else
  note: If Condition
  cmdPower : Inport
  Power : Inport  Port=2
  Action Port : ActionPort
  If : If  IfExpression=u1 >= 50
  Merge : Merge
  Merge1 : Merge
  power else : Subsystem  TreatAsAtomicUnit=on
  power if : Subsystem  TreatAsAtomicUnit=on
  T : Outport  VectorParamsAs1DForOutWhenUnconnected=off
  P2 : Outport  Port=2  VectorParamsAs1DForOutWhenUnconnected=off
  wires:
  cmdPower/1 -> [cmdPower]
  Power/1 -> [Power]
  [Power] -> If/1
  If/1 -> [if]
  If/2 -> [else]
  [if] -> power if/Action
  [else] -> power else/Action
  [cmdPower] -> power if/1(cmdPower)
  Merge/1 -> T/1
  Merge1/1 -> P2/1
  power if/1(T) -> Merge/1
  power else/2(P2) -> Merge1/2
  power else/1(T) -> Merge/2
  power if/2(P2) -> Merge1/1
  [Power] -> power else/1(Power)

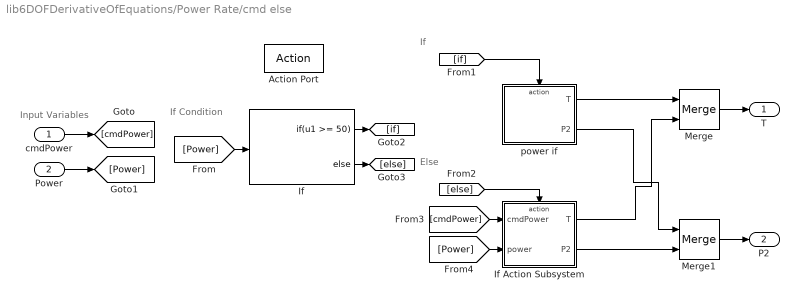
== system lib6DOFDerivativeOfEquations/Power Rate/cmd else ==
  note: If
  note: Else
  note: Input Variables
  note: If Condition
  cmdPower : Inport
  Power : Inport  Port=2
  Action Port : ActionPort
  If : If  IfExpression=u1 >= 50
  If Action Subsystem : Subsystem  TreatAsAtomicUnit=on
  Merge : Merge
  Merge1 : Merge
  power if : Subsystem  TreatAsAtomicUnit=on
  T : Outport  VectorParamsAs1DForOutWhenUnconnected=off
  P2 : Outport  Port=2  VectorParamsAs1DForOutWhenUnconnected=off
  wires:
  cmdPower/1 -> [cmdPower]
  Power/1 -> [Power]
  [Power] -> If/1
  If/1 -> [if]
  If/2 -> [else]
  [if] -> power if/Action
  [else] -> If Action Subsystem/Action
  [cmdPower] -> If Action Subsystem/1(cmdPower)
  [Power] -> If Action Subsystem/2(power)
  power if/2(P2) -> Merge1/1
  If Action Subsystem/1(T) -> Merge/2
  Merge1/1 -> P2/1
  If Action Subsystem/2(P2) -> Merge1/2
  power if/1(T) -> Merge/1
  Merge/1 -> T/1

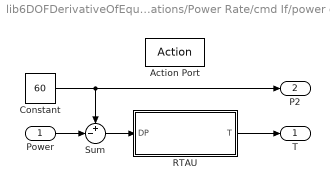
== system lib6DOFDerivativeOfEquations/Power Rate/cmd If/power else ==
  Power : Inport
  Action Port : ActionPort
  Constant : Constant  Value=60
  RTAU : Subsystem
  Sum : Sum  Inputs=+-|
  T : Outport  VectorParamsAs1DForOutWhenUnconnected=off
  P2 : Outport  Port=2  VectorParamsAs1DForOutWhenUnconnected=off
  wires:
  Power/1 -> Sum/2
  RTAU/1(T) -> T/1
  Constant/1 -> Sum/1, P2/1
  Sum/1 -> RTAU/1(DP)

== system lib6DOFDerivativeOfEquations/Power Rate/cmd If/power if ==
  cmdPower : Inport
  Action Port : ActionPort
  Constant : Constant  Value=5
  T : Outport  VectorParamsAs1DForOutWhenUnconnected=off
  P2 : Outport  Port=2  VectorParamsAs1DForOutWhenUnconnected=off
  wires:
  cmdPower/1 -> P2/1
  Constant/1 -> T/1

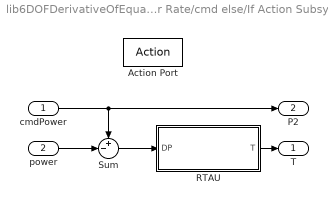
== system lib6DOFDerivativeOfEquations/Power Rate/cmd else/If Action Subsystem ==
  cmdPower : Inport
  power : Inport  Port=2
  Action Port : ActionPort
  RTAU : Subsystem
  Sum : Sum  Inputs=+-|
  T : Outport  VectorParamsAs1DForOutWhenUnconnected=off
  P2 : Outport  Port=2  VectorParamsAs1DForOutWhenUnconnected=off
  wires:
  power/1 -> Sum/2
  cmdPower/1 -> Sum/1, P2/1
  RTAU/1(T) -> T/1
  Sum/1 -> RTAU/1(DP)

== system lib6DOFDerivativeOfEquations/Power Rate/cmd else/power if ==
  Action Port : ActionPort
  Constant : Constant  Value=5
  Constant1 : Constant  Value=40
  T : Outport  VectorParamsAs1DForOutWhenUnconnected=off
  P2 : Outport  Port=2  VectorParamsAs1DForOutWhenUnconnected=off
  wires:
  Constant/1 -> T/1
  Constant1/1 -> P2/1

== system lib6DOFDerivativeOfEquations/Power Rate/cmd If/power else/RTAU ==
  DP : Inport
  If : If  IfExpression=u1 <= 25  ElseIfExpressions=u1 >= 50
  If Action Subsystem : Subsystem  TreatAsAtomicUnit=on
  If Action Subsystem1 : Subsystem  TreatAsAtomicUnit=on
  If Action Subsystem2 : Subsystem  TreatAsAtomicUnit=on
  Merge : Merge  Inputs=3
  T : Outport  VectorParamsAs1DForOutWhenUnconnected=off
  wires:
  DP/1 -> If Action Subsystem2/1(DP), If/1
  If/2 -> If Action Subsystem1/Action
  If/1 -> If Action Subsystem/Action
  If/3 -> If Action Subsystem2/Action
  If Action Subsystem/1(T) -> Merge/1
  If Action Subsystem1/1(T) -> Merge/2
  If Action Subsystem2/1(T) -> Merge/3
  Merge/1 -> T/1

== system lib6DOFDerivativeOfEquations/Power Rate/cmd else/If Action Subsystem/RTAU ==
  DP : Inport
  If : If  IfExpression=u1 <= 25  ElseIfExpressions=u1 >= 50
  If Action Subsystem : Subsystem  TreatAsAtomicUnit=on
  If Action Subsystem1 : Subsystem  TreatAsAtomicUnit=on
  If Action Subsystem2 : Subsystem  TreatAsAtomicUnit=on
  Merge : Merge  Inputs=3
  T : Outport  VectorParamsAs1DForOutWhenUnconnected=off
  wires:
  Merge/1 -> T/1
  If Action Subsystem2/1(T) -> Merge/3
  If Action Subsystem1/1(T) -> Merge/2
  If Action Subsystem/1(T) -> Merge/1
  If/3 -> If Action Subsystem2/Action
  If/1 -> If Action Subsystem/Action
  If/2 -> If Action Subsystem1/Action
  DP/1 -> If/1, If Action Subsystem2/1(DP)

== system lib6DOFDerivativeOfEquations/Power Rate/cmd If/power else/RTAU/If Action Subsystem ==
  Action Port : ActionPort
  Constant : Constant
  T : Outport  VectorParamsAs1DForOutWhenUnconnected=off
  wires:
  Constant/1 -> T/1

== system lib6DOFDerivativeOfEquations/Power Rate/cmd If/power else/RTAU/If Action Subsystem1 ==
  Action Port : ActionPort
  Constant : Constant  Value=0.1
  T : Outport  VectorParamsAs1DForOutWhenUnconnected=off
  wires:
  Constant/1 -> T/1

== system lib6DOFDerivativeOfEquations/Power Rate/cmd If/power else/RTAU/If Action Subsystem2 ==
  DP : Inport
  Action Port : ActionPort
  Constant : Constant  Value=1.9
  Gain : Gain  Gain=0.036
  Sum : Sum  Inputs=|-+
  T : Outport  VectorParamsAs1DForOutWhenUnconnected=off
  wires:
  DP/1 -> Gain/1
  Gain/1 -> Sum/1
  Sum/1 -> T/1
  Constant/1 -> Sum/2

== system lib6DOFDerivativeOfEquations/Power Rate/cmd else/If Action Subsystem/RTAU/If Action Subsystem ==
  Action Port : ActionPort
  Constant : Constant
  T : Outport  VectorParamsAs1DForOutWhenUnconnected=off
  wires:
  Constant/1 -> T/1

== system lib6DOFDerivativeOfEquations/Power Rate/cmd else/If Action Subsystem/RTAU/If Action Subsystem1 ==
  Action Port : ActionPort
  Constant : Constant  Value=0.1
  T : Outport  VectorParamsAs1DForOutWhenUnconnected=off
  wires:
  Constant/1 -> T/1

== system lib6DOFDerivativeOfEquations/Power Rate/cmd else/If Action Subsystem/RTAU/If Action Subsystem2 ==
  DP : Inport
  Action Port : ActionPort
  Constant : Constant  Value=1.9
  Gain : Gain  Gain=0.036
  Sum : Sum  Inputs=|-+
  T : Outport  VectorParamsAs1DForOutWhenUnconnected=off
  wires:
  Constant/1 -> Sum/2
  Sum/1 -> T/1
  Gain/1 -> Sum/1
  DP/1 -> Gain/1
